simulink model "RCmodel"  (R2023a)
settings: Solver=FixedStepAuto  StartTime=0.0  StopTime=90698  FixedStep=1  RelTol=1e-3

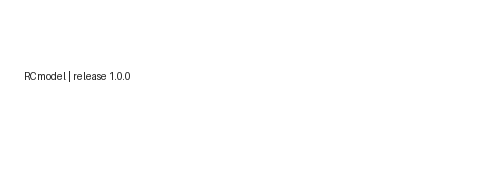
[thumbnail: Simulink's stored preview of the top-level diagram]
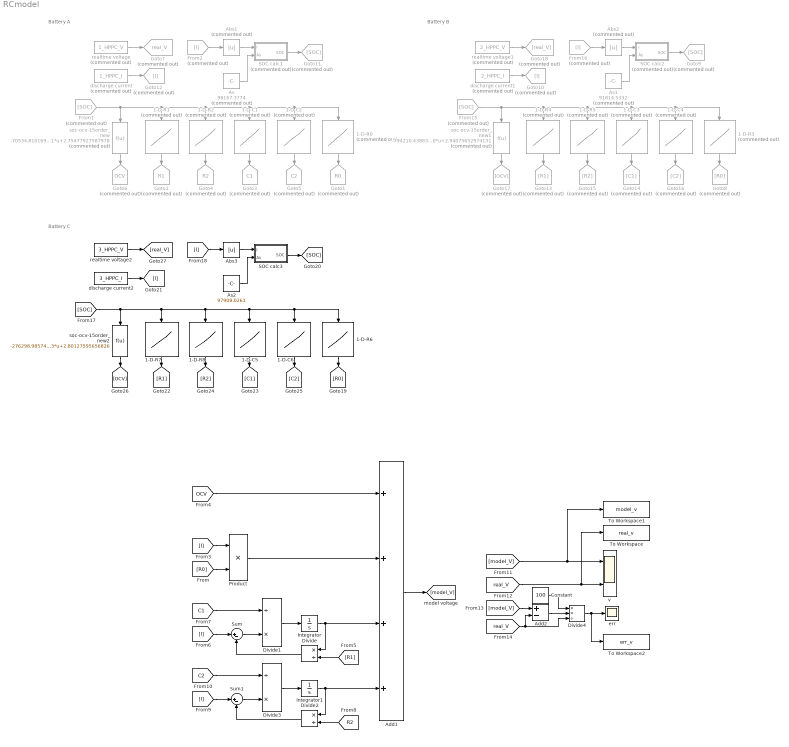
== system RCmodel ==
  note: Battery A
  note: Battery B
  note: Battery C
  1-D-C1 : Lookup_n-D  Commented=on  NumberOfTableDimensions=1  BreakpointsForDimension1=[-1.77E-15, 0.037269293, 0.083116861, 0.128963973, 0.174807506, 0.220651377, 0.266495278, 0.312338437, 0.358182054, 0.40402557, 0.449869074, 0.495712509, 0.541556044, 0.587400025, 0.633243688, 0.679087252, 0.724930767, 0.770773292, 0.816616177, 0.8624587, 0.908303278, 0.954151828]  Table=[4384.105654, 9231.940513, 11088.72237, 15403.93995, 18455.27759, 22262.89883, 18250.89605, 25235.00938, 19703.41311, 20930.29445, 17424.20855, 19725.2804, 21066.30228, 26715.94609, 24673.77168, 45424.65176, 28463.93232, 19061.93163, 15685.57933, 14799.5027, 32105.98505, 26182.43606]  InternalRulePriority=Speed  RndMeth=Simplest
  1-D-C2 : Lookup_n-D  Commented=on  NumberOfTableDimensions=1  BreakpointsForDimension1=[-1.77E-15, 0.037269293, 0.083116861, 0.128963973, 0.174807506, 0.220651377, 0.266495278, 0.312338437, 0.358182054, 0.40402557, 0.449869074, 0.495712509, 0.541556044, 0.587400025, 0.633243688, 0.679087252, 0.724930767, 0.770773292, 0.816616177, 0.8624587, 0.908303278, 0.954151828]  Table=[128457.3479, 465470.6122, 495152.4038, 743899.8473, 723042.0864, 811858.4125, 406573.4995, 454452.6409, 480505.5618, 704377.8381, 645807.3163, 845882.7961, 864024.0546, 832452.6584, 413783.5189, 382952.2768, 796906.3219, 832059.7725, 799062.2851, 723078.4735, 1813924.946, 1387381.585]  InternalRulePriority=Speed  RndMeth=Simplest
  1-D-C3 : Lookup_n-D  Commented=on  NumberOfTableDimensions=1  BreakpointsForDimension1=[-7.8419E-08, 0.019714291, 0.068728061, 0.117742026, 0.166756071, 0.21576937, 0.264783571, 0.313798204, 0.362812366, 0.411826096, 0.460839905, 0.50985442, 0.55886819, 0.60788247, 0.656896828, 0.705911421, 0.754926406, 0.803941313, 0.852956063, 0.901970617, 0.950985446]  Table=[225214.1434, 187025.2766, 296294.3583, 325129.1549, 382794.7295, 371710.2995, 353976.6676, 381282.3938, 488296.3231, 462238.5316, 712185.7898, 891276.2929, 786232.5864, 455006.0004, 322811.3497, 309379.8901, 321116.448, 741388.8307, 942394.5955, 1060535.922, 1063695.943]  InternalRulePriority=Speed  RndMeth=Simplest
  1-D-C4 : Lookup_n-D  Commented=on  NumberOfTableDimensions=1  BreakpointsForDimension1=[-7.8419E-08, 0.019714291, 0.068728061, 0.117742026, 0.166756071, 0.21576937, 0.264783571, 0.313798204, 0.362812366, 0.411826096, 0.460839905, 0.50985442, 0.55886819, 0.60788247, 0.656896828, 0.705911421, 0.754926406, 0.803941313, 0.852956063, 0.901970617, 0.950985446]  Table=[1671.127633, 1673.968389, 4565.243665, 6209.535618, 11242.6131, 9787.657058, 11449.06044, 14014.79555, 15699.36024, 13663.69917, 14717.09328, 14685.37445, 16462.66037, 11898.52641, 12704.67604, 16178.70649, 18177.54925, 20734.64693, 17610.56739, 15941.06135, 15784.62672]  InternalRulePriority=Speed  RndMeth=Simplest
  1-D-C5 : Lookup_n-D  NumberOfTableDimensions=1  BreakpointsForDimension1=[2.9109E-07, 0.034704903, 0.080678392, 0.126651918, 0.172626069, 0.218599963, 0.264561539, 0.310535727, 0.35649723, 0.402458916, 0.448432994, 0.494395195, 0.540356772, 0.586318863, 0.632281101, 0.678243265, 0.724205797, 0.770168256, 0.81613042, 0.862092732, 0.908054492, 0.954027467]  Table=[148211.7874, 379943.691, 507178.8648, 540877.9099, 565031.5977, 599113.5276, 468851.5567, 439228.3613, 564632.19, 525250.0917, 713932.6032, 938377.816, 623343.6413, 597265.7355, 374444.1491, 318686.1875, 638311.9656, 790877.9592, 883896.1639, 825362.4483, 795349.2136, 1510862.771]  InternalRulePriority=Speed  RndMeth=Simplest
  1-D-C6 : Lookup_n-D  NumberOfTableDimensions=1  BreakpointsForDimension1=[2.9109E-07, 0.034704903, 0.080678392, 0.126651918, 0.172626069, 0.218599963, 0.264561539, 0.310535727, 0.35649723, 0.402458916, 0.448432994, 0.494395195, 0.540356772, 0.586318863, 0.632281101, 0.678243265, 0.724205797, 0.770168256, 0.81613042, 0.862092732, 0.908054492, 0.954027467]  Table=[2196.493417, 6254.414395, 10027.09575, 11640.94595, 15150.56735, 14939.39571, 22277.23726, 21788.57636, 21198.25628, 16155.2285, 17423.71863, 20324.46195, 14880.37747, 17370.84513, 17908.76661, 37791.77026, 30450.72328, 20196.6933, 17282.88891, 15011.20802, 15927.09163, 25703.81768]  InternalRulePriority=Speed  RndMeth=Simplest
  1-D-R0 : Lookup_n-D  Commented=on  NumberOfTableDimensions=1  BreakpointsForDimension1=[-1.77E-15, 0.037269293, 0.083116861, 0.128963973, 0.174807506, 0.220651377, 0.266495278, 0.312338437, 0.358182054, 0.40402557, 0.449869074, 0.495712509, 0.541556044, 0.587400025, 0.633243688, 0.679087252, 0.724930767, 0.770773292, 0.816616177, 0.8624587, 0.908303278, 0.954151828]  Table=[0.002377198, 0.001865386, 0.001636924, 0.00171298, 0.001637029, 0.001565196, 0.001560989, 0.001564868, 0.001565063, 0.001489024, 0.00148912, 0.001489024, 0.001488935, 0.00148912, 0.001560989, 0.00148884, 0.001489209, 0.001416902, 0.001340922, 0.001412783, 0.001565063, 0.001560894]  InternalRulePriority=Speed  RndMeth=Simplest
  1-D-R1 : Lookup_n-D  Commented=on  NumberOfTableDimensions=1  BreakpointsForDimension1=[-1.77E-15, 0.037269293, 0.083116861, 0.128963973, 0.174807506, 0.220651377, 0.266495278, 0.312338437, 0.358182054, 0.40402557, 0.449869074, 0.495712509, 0.541556044, 0.587400025, 0.633243688, 0.679087252, 0.724930767, 0.770773292, 0.816616177, 0.8624587, 0.908303278, 0.954151828]  Table=[0.008529593, 0.004641446, 0.003726801, 0.002802356, 0.002708475, 0.002378808, 0.002151212, 0.002286208, 0.002397823, 0.002284936, 0.002097119, 0.001946165, 0.001814466, 0.001701571, 0.001733472, 0.002128072, 0.002614288, 0.00242572, 0.002193873, 0.001943976, 0.001716154, 0.001577034]  InternalRulePriority=Speed  RndMeth=Simplest
  1-D-R2 : Lookup_n-D  Commented=on  NumberOfTableDimensions=1  BreakpointsForDimension1=[-1.77E-15, 0.037269293, 0.083116861, 0.128963973, 0.174807506, 0.220651377, 0.266495278, 0.312338437, 0.358182054, 0.40402557, 0.449869074, 0.495712509, 0.541556044, 0.587400025, 0.633243688, 0.679087252, 0.724930767, 0.770773292, 0.816616177, 0.8624587, 0.908303278, 0.954151828]  Table=[0.008096678, 0.002514972, 0.001860654, 0.001787177, 0.001528518, 0.001475616, 0.001899763, 0.002008577, 0.001743754, 0.001436378, 0.001334078, 0.001264856, 0.001252993, 0.001381405, 0.00278871, 0.002181145, 0.001385783, 0.001223234, 0.001136039, 0.001078898, 0.000787639, 0.000892343]  InternalRulePriority=Speed  RndMeth=Simplest
  1-D-R3 : Lookup_n-D  Commented=on  NumberOfTableDimensions=1  BreakpointsForDimension1=[-7.8419E-08, 0.019714291, 0.068728061, 0.117742026, 0.166756071, 0.21576937, 0.264783571, 0.313798204, 0.362812366, 0.411826096, 0.460839905, 0.50985442, 0.55886819, 0.60788247, 0.656896828, 0.705911421, 0.754926406, 0.803941313, 0.852956063, 0.901970617, 0.950985446]  Table=[0.005142418, 0.004920407, 0.004844512, 0.004848168, 0.00477236, 0.004844207, 0.004916611, 0.004768351, 0.004768354, 0.004767743, 0.004920582, 0.00484046, 0.004695644, 0.004619808, 0.004547664, 0.004543704, 0.004467293, 0.004547664, 0.004547368, 0.004399462, 0.004246964]  InternalRulePriority=Speed  RndMeth=Simplest
  1-D-R4 : Lookup_n-D  Commented=on  NumberOfTableDimensions=1  BreakpointsForDimension1=[-7.8419E-08, 0.019714291, 0.068728061, 0.117742026, 0.166756071, 0.21576937, 0.264783571, 0.313798204, 0.362812366, 0.411826096, 0.460839905, 0.50985442, 0.55886819, 0.60788247, 0.656896828, 0.705911421, 0.754926406, 0.803941313, 0.852956063, 0.901970617, 0.950985446]  Table=[0.00461437, 0.004542772, 0.002927848, 0.002489007, 0.00261231, 0.002854022, 0.002839665, 0.002705643, 0.002322517, 0.001930102, 0.001569536, 0.001434529, 0.001559029, 0.002338951, 0.003742684, 0.00311492, 0.00238201, 0.001540864, 0.001263662, 0.001122294, 0.001006783]  InternalRulePriority=Speed  RndMeth=Simplest
  1-D-R5 : Lookup_n-D  Commented=on  NumberOfTableDimensions=1  BreakpointsForDimension1=[-7.8419E-08, 0.019714291, 0.068728061, 0.117742026, 0.166756071, 0.21576937, 0.264783571, 0.313798204, 0.362812366, 0.411826096, 0.460839905, 0.50985442, 0.55886819, 0.60788247, 0.656896828, 0.705911421, 0.754926406, 0.803941313, 0.852956063, 0.901970617, 0.950985446]  Table=[0.022805443, 0.021704309, 0.009347226, 0.005943316, 0.004810936, 0.004550218, 0.004093036, 0.003809411, 0.003763955, 0.003626777, 0.003515244, 0.003368593, 0.002718876, 0.003041587, 0.003017746, 0.002947958, 0.003081328, 0.00338066, 0.003232809, 0.003004131, 0.002690434]  InternalRulePriority=Speed  RndMeth=Simplest
  1-D-R6 : Lookup_n-D  NumberOfTableDimensions=1  BreakpointsForDimension1=[2.9109E-07, 0.034704903, 0.080678392, 0.126651918, 0.172626069, 0.218599963, 0.264561539, 0.310535727, 0.35649723, 0.402458916, 0.448432994, 0.494395195, 0.540356772, 0.586318863, 0.632281101, 0.678243265, 0.724205797, 0.770168256, 0.81613042, 0.862092732, 0.908054492, 0.954027467]  Table=[0.002528647, 0.001936736, 0.001933092, 0.002009272, 0.001857034, 0.001932965, 0.001937093, 0.001860779, 0.001865146, 0.001940916, 0.001785007, 0.001860795, 0.001784893, 0.001792897, 0.001860957, 0.001860919, 0.001788901, 0.0017849, 0.001708766, 0.001708843, 0.001636824, 0.001636826]  InternalRulePriority=Speed  RndMeth=Simplest
  1-D-R7 : Lookup_n-D  NumberOfTableDimensions=1  BreakpointsForDimension1=[2.9109E-07, 0.034704903, 0.080678392, 0.126651918, 0.172626069, 0.218599963, 0.264561539, 0.310535727, 0.35649723, 0.402458916, 0.448432994, 0.494395195, 0.540356772, 0.586318863, 0.632281101, 0.678243265, 0.724205797, 0.770168256, 0.81613042, 0.862092732, 0.908054492, 0.954027467]  Table=[0.007426917, 0.002725754, 0.002056684, 0.002051955, 0.001788462, 0.001933155, 0.002069724, 0.00225684, 0.001884435, 0.0016594, 0.001488249, 0.001395496, 0.001419538, 0.001566898, 0.002844649, 0.002781912, 0.001682693, 0.00138196, 0.001233272, 0.001177427, 0.001101257, 0.000924041]  InternalRulePriority=Speed  RndMeth=Simplest
  1-D-R8 : Lookup_n-D  NumberOfTableDimensions=1  BreakpointsForDimension1=[2.9109E-07, 0.034704903, 0.080678392, 0.126651918, 0.172626069, 0.218599963, 0.264561539, 0.310535727, 0.35649723, 0.402458916, 0.448432994, 0.494395195, 0.540356772, 0.586318863, 0.632281101, 0.678243265, 0.724205797, 0.770168256, 0.81613042, 0.862092732, 0.908054492, 0.954027467]  Table=[0.012678994, 0.006218342, 0.004585322, 0.003481865, 0.003212414, 0.002922909, 0.002535113, 0.002663285, 0.002728817, 0.002644002, 0.002455207, 0.0022745, 0.002186381, 0.002057863, 0.001998786, 0.002105164, 0.002862673, 0.002808045, 0.002531815, 0.002274687, 0.00198128, 0.001756841]  InternalRulePriority=Speed  RndMeth=Simplest
  Abs1 : Abs  Commented=on  SaturateOnIntegerOverflow=off
  Abs2 : Abs  Commented=on  SaturateOnIntegerOverflow=off
  Abs3 : Abs  SaturateOnIntegerOverflow=off
  Add1 : Sum  Inputs=++++
  Add2 : Sum  Inputs=+-
  As : Constant  Commented=on  Value=98167.3774
  As1 : Constant  Commented=on  Value=91814.5332
  As2 : Constant  Value=97908.0261
  Constant : Constant  Value=100
  Divide : Product  Inputs=*/
  Divide1 : Product  Inputs=/*
  Divide2 : Product  Inputs=*/
  Divide3 : Product  Inputs=/*
  Divide4 : Product  Inputs=**/
  From1 : From  Commented=on  GotoTag=SOC
  From15 : From  Commented=on  GotoTag=SOC
  From16 : From  Commented=on  GotoTag=I
  From2 : From  Commented=on  GotoTag=I
  Goto1 : Goto  Commented=on  GotoTag=R0  TagVisibility=global
  Goto10 : Goto  Commented=on  GotoTag=I
  Goto11 : Goto  Commented=on  GotoTag=SOC
  Goto12 : Goto  Commented=on  GotoTag=I
  Goto13 : Goto  Commented=on  GotoTag=R1
  Goto14 : Goto  Commented=on  GotoTag=C1
  Goto15 : Goto  Commented=on  GotoTag=R2
  Goto16 : Goto  Commented=on  GotoTag=C2
  Goto17 : Goto  Commented=on  GotoTag=OCV
  Goto18 : Goto  Commented=on  GotoTag=real_V
  Goto2 : Goto  Commented=on  GotoTag=R1  TagVisibility=global
  Goto3 : Goto  Commented=on  GotoTag=C1  TagVisibility=global
  Goto4 : Goto  Commented=on  GotoTag=R2  TagVisibility=global
  Goto5 : Goto  Commented=on  GotoTag=C2  TagVisibility=global
  Goto6 : Goto  Commented=on  GotoTag=OCV  TagVisibility=global
  Goto7 : Goto  Commented=on  GotoTag=real_V  TagVisibility=global
  Goto8 : Goto  Commented=on  GotoTag=R0
  Goto9 : Goto  Commented=on  GotoTag=SOC
  Integrator : Integrator
  Integrator1 : Integrator
  Product : Product
  SOC calc1 : Subsystem  Commented=on
  SOC calc2 : Subsystem  Commented=on
  SOC calc3 : Subsystem
  Sum : Sum  Inputs=|+-
  Sum1 : Sum  Inputs=|+-
  To Workspace : ToWorkspace  VariableName=real_v  SaveFormat=Timeseries  SampleTime=-1
  To Workspace1 : ToWorkspace  VariableName=model_v  SaveFormat=Timeseries  SampleTime=-1
  To Workspace2 : ToWorkspace  VariableName=err_v  SaveFormat=Timeseries  SampleTime=-1
  discharge current : FromFile  Commented=on  FileName=1_HPPC_I  SampleTime=0
  discharge current1 : FromFile  Commented=on  FileName=2_HPPC_I  SampleTime=0
  discharge current2 : FromFile  FileName=3_HPPC_I  SampleTime=0
  err : Scope
  realtime voltage : FromFile  Commented=on  FileName=1_HPPC_V  SampleTime=0
  realtime voltage1 : FromFile  Commented=on  FileName=2_HPPC_V  SampleTime=0
  realtime voltage2 : FromFile  FileName=3_HPPC_V  SampleTime=0
  soc-ocv-15order_new : Fcn  Commented=on  Expr=-70534.8101697033*u^15+667631.040368181*u^14-2808879.23048057*u^13+6966732.70412309*u^12-11358348.0257989*u^11+12823791.8442839*u^10-10271539.9511109*u^9+5870162.95223606*u^8-2366653.89631967*u^7+650005.644269369*u^6-111485.470420124*u^5+8763.85610880856*u^4+518.950645240942*u^3-179.924509925818*u^2+14.9938870907751*u+2.75477927587978
  soc-ocv-15order_new1 : Fcn  Commented=on  Expr=-794210.438834610*u^15+5987745.61568300*u^14-20439836.7898101*u^13+41772168.8258101*u^12-56921777.5690841*u^11+54490938.0492044*u^10-37586563.2858994*u^9+18834958.2927790*u^8-6814558.32935900*u^7+1740625.65248685*u^6-299189.844437199*u^5+31109.3414812153*u^4-1360.69378520401*u^3-57.0272510664786*u^2+8.63635391828670*u+2.94075652974131
  soc-ocv-15order_new2 : Fcn  Expr=-276298.985749310*u^15+2079100.19510310*u^14-7146107.09932892*u^13+14857923.9617195*u^12-20833240.2231729*u^11+20756759.1140984*u^10-15054210.4175051*u^9+7991543.21304879*u^8-3070959.05248522*u^7+827625.466792177*u^6-145769.880033493*u^5+13780.6338711194*u^4-19.7560716602156*u^3-139.705484335419*u^2+13.1062128117163*u+2.80127595656826
  v : Scope  NumInputPorts=2
  wires:
  [model_V] -> v/1, To Workspace1/1
  Divide3/1 -> Integrator1/1
  Divide4/1 -> To Workspace2/1, err/1
  [I] -> Sum/1
  [I] -> Sum1/1
  [model_V] -> Add2/1
  Divide/1 -> Sum/2
  [R2] -> Divide2/2
  [C2] -> Divide3/1
  [OCV] -> Add1/1
  [R0] -> Product/2
  Integrator1/1 -> Divide2/1, Add1/4
  Sum/1 -> Divide1/2
  Divide2/1 -> Sum1/2
  [real_V] -> To Workspace/1, v/2
  [real_V] -> Divide4/3, Add2/2
  [R1] -> Divide/2
  Divide1/1 -> Integrator/1
  Add1/1 -> [model_V]
  [I] -> Product/1
  Sum1/1 -> Divide3/2
  Product/1 -> Add1/2
  Add2/1 -> Divide4/2
  [C1] -> Divide1/1
  Constant/1 -> Divide4/1
  Integrator/1 -> Divide/1, Add1/3
  1-D-C2/1 -> Goto5/1
  As/1 -> SOC calc1/2(As)
  1-D-R0/1 -> Goto1/1
  realtime voltage/1 -> Goto7/1
  SOC calc1/1(SOC) -> Goto11/1
  1-D-C1/1 -> Goto3/1
  From2/1 -> Abs1/1
  From1/1 -> 1-D-R0/1, 1-D-C2/1, 1-D-C1/1, 1-D-R2/1, 1-D-R1/1, soc-ocv-15order_new/1
  1-D-R2/1 -> Goto4/1
  Abs1/1 -> SOC calc1/1(I)
  discharge current/1 -> Goto12/1
  soc-ocv-15order_new/1 -> Goto6/1
  1-D-R1/1 -> Goto2/1
  soc-ocv-15order_new1/1 -> Goto17/1
  1-D-R3/1 -> Goto8/1
  Abs2/1 -> SOC calc2/1(I)
  As1/1 -> SOC calc2/2(As)
  SOC calc2/1(SOC) -> Goto9/1
  realtime voltage1/1 -> Goto18/1
  1-D-C3/1 -> Goto14/1
  1-D-C4/1 -> Goto16/1
  1-D-R4/1 -> Goto13/1
  discharge current1/1 -> Goto10/1
  From16/1 -> Abs2/1
  1-D-R5/1 -> Goto15/1
  From15/1 -> 1-D-R3/1, 1-D-C4/1, 1-D-C3/1, 1-D-R5/1, 1-D-R4/1, soc-ocv-15order_new1/1
  Abs3/1 -> SOC calc3/1(I)
  1-D-C6/1 -> [C2]
  As2/1 -> SOC calc3/2(As)
  1-D-R6/1 -> [R0]
  realtime voltage2/1 -> [real_V]
  [I] -> Abs3/1
  1-D-R7/1 -> [R1]
  [SOC] -> 1-D-R6/1, 1-D-C6/1, 1-D-C5/1, 1-D-R8/1, 1-D-R7/1, soc-ocv-15order_new2/1
  soc-ocv-15order_new2/1 -> [OCV]
  1-D-C5/1 -> [C1]
  discharge current2/1 -> [I]
  1-D-R8/1 -> [R2]
  SOC calc3/1(SOC) -> [SOC]

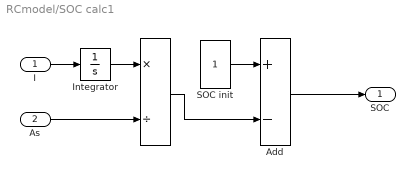
== system RCmodel/SOC calc1 ==
  I : Inport
  As : Inport  Port=2
  "     " : Product  Inputs=*/
  Add : Sum  Inputs=+-
  Integrator : Integrator
  SOC init : Constant
  SOC : Outport  VectorParamsAs1DForOutWhenUnconnected=off
  wires:
  Add/1 -> SOC/1
  SOC init/1 -> Add/1
  I/1 -> Integrator/1
  Integrator/1 -> "     "/1
  "     "/1 -> Add/2
  As/1 -> "     "/2

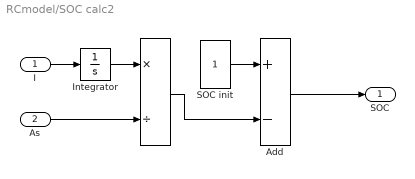
== system RCmodel/SOC calc2 ==
  I : Inport
  As : Inport  Port=2
  "     " : Product  Inputs=*/
  Add : Sum  Inputs=+-
  Integrator : Integrator
  SOC init : Constant
  SOC : Outport  VectorParamsAs1DForOutWhenUnconnected=off
  wires:
  Add/1 -> SOC/1
  SOC init/1 -> Add/1
  I/1 -> Integrator/1
  Integrator/1 -> "     "/1
  "     "/1 -> Add/2
  As/1 -> "     "/2

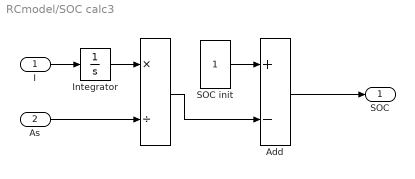
== system RCmodel/SOC calc3 ==
  I : Inport
  As : Inport  Port=2
  "     " : Product  Inputs=*/
  Add : Sum  Inputs=+-
  Integrator : Integrator
  SOC init : Constant
  SOC : Outport  VectorParamsAs1DForOutWhenUnconnected=off
  wires:
  Add/1 -> SOC/1
  SOC init/1 -> Add/1
  I/1 -> Integrator/1
  Integrator/1 -> "     "/1
  "     "/1 -> Add/2
  As/1 -> "     "/2
